simulink model "Hvac_control"  (R2021a)
settings: Solver=ode45  StartTime=0  StopTime=Tf  FixedStep=Ts  RelTol=1e-3
values from neighbouring files (symbols this model uses):
  b = []    [control_predictivo.m]
  Ts = 600    [p2.m]
undefined symbols (not defined in the file or in its folder): a, g
libraries: simulink x2
settings Model: Creator=rober  LastModifiedBy=sebag
settings SolverCC: AlgebraicLoopSolver=TrustRegion
settings DataIOCC: ReturnWorkspaceOutputs=off
settings OptimizationCC: LifeSpan=inf
settings DebuggingCC: SFMachineParentedDataDiag=warning  ArithmeticOperatorsInVariantConditions=warning
settings SFSimCC: CustomCodeUndefinedFunction=UseInterfaceOnly
settings CodeAppCC: StateflowObjectComments=on

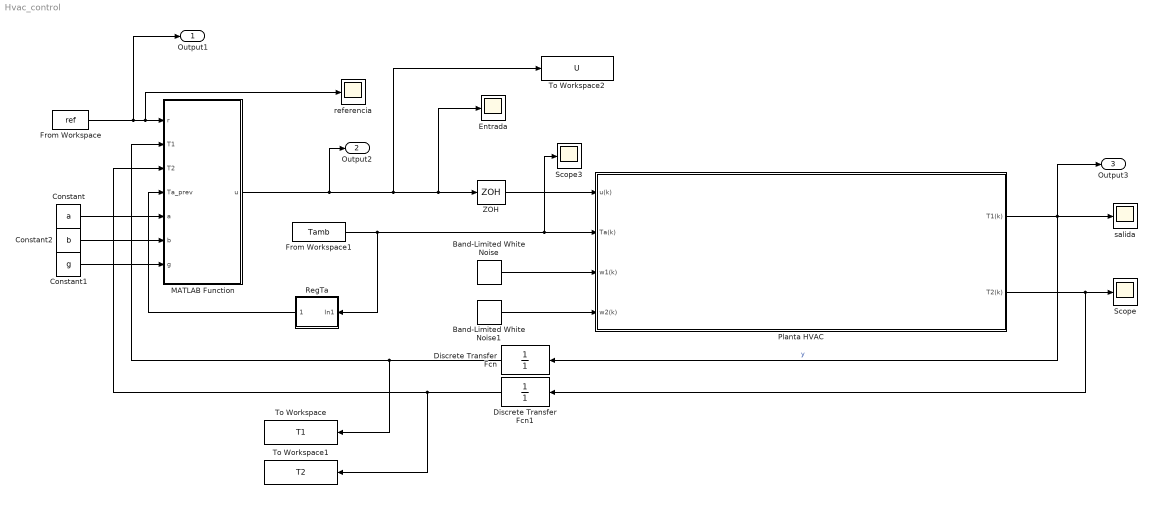
== system Hvac_control ==
  Band-Limited White Noise : simulink/Sources/Band-Limited White Noise  Cov=[0.001]  Ts=Ts  seed=[23341]
  Band-Limited White Noise1 : simulink/Sources/Band-Limited White Noise  Cov=[0.001]  Ts=Ts  seed=[23341]
  Constant : Constant  Value=a
  Constant1 : Constant  Value=g
  Constant2 : Constant  Value=b
  Discrete Transfer Fcn : DiscreteTransferFcn  Denominator=[1]  SampleTime=Ts
  Discrete Transfer Fcn1 : DiscreteTransferFcn  Denominator=[1]  SampleTime=Ts
  Entrada : Scope
  From Workspace : FromWorkspace  VariableName=ref  SampleTime=Ts
  From Workspace1 : FromWorkspace  VariableName=Tamb
  MATLAB Function : MATLAB Function  TreatAsAtomicUnit=on
  Planta HVAC : Subsystem
      mask Display: image('Planta_HVAC.jpg')
  RegTa : Subsystem
  Scope : Scope
  Scope3 : Scope
  To Workspace : ToWorkspace  VariableName=T1  SampleTime=-1
      settings: Save2DSignal=2-D array (concatenate along first dimension)
  To Workspace1 : ToWorkspace  VariableName=T2  SampleTime=Ts
      settings: Save2DSignal=2-D array (concatenate along first dimension)
  To Workspace2 : ToWorkspace  VariableName=U  SampleTime=Ts
      settings: Save2DSignal=2-D array (concatenate along first dimension)
  ZOH : ZeroOrderHold  SampleTime=-1
  referencia : Scope
  salida : Scope
  Output1 : Outport  SignalName=ref
  Output2 : Outport  Port=2  SignalName=u  PortDimensions=[1]
  Output3 : Outport  Port=3  SignalName=y  PortDimensions=[1]
  wires:
  From Workspace1/1 -> Scope3/1, Planta HVAC/2(Ta(k)), RegTa/1(In1)
  Band-Limited White Noise/1 -> Planta HVAC/3(w1(k))
  Band-Limited White Noise1/1 -> Planta HVAC/4(w2(k))
  From Workspace/1 -> Output1/1, referencia/1, MATLAB Function/1(r)
  Planta HVAC/2(T2(k)) -> Discrete Transfer Fcn1/1, Scope/1
  RegTa/1(Ta_prev) -> MATLAB Function/4(Ta_prev)
  Planta HVAC/1(T1(k)) -> Discrete Transfer Fcn/1, salida/1, Output3/1  "y"
  Discrete Transfer Fcn1/1 -> To Workspace1/1, MATLAB Function/3(T2)
  Discrete Transfer Fcn/1 -> MATLAB Function/2(T1), To Workspace/1
  Constant/1 -> MATLAB Function/5(a)
  Constant1/1 -> MATLAB Function/7(g)
  Constant2/1 -> MATLAB Function/6(b)
  MATLAB Function/1(u) -> To Workspace2/1, Entrada/1, ZOH/1, Output2/1
  ZOH/1 -> Planta HVAC/1(u(k))

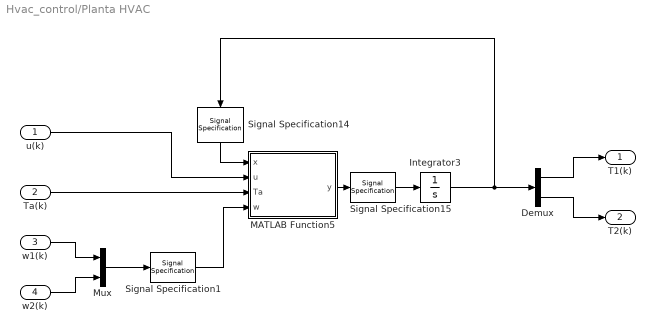
== system Hvac_control/Planta HVAC ==
  u(k) : Inport
  Ta(k) : Inport  Port=2
  w1(k) : Inport  Port=3
  w2(k) : Inport  Port=4
  Demux : Demux  Outputs=2
  Integrator3 : Integrator  InitialCondition=[10.12;10.12]
  MATLAB Function5 : MATLAB Function  TreatAsAtomicUnit=on
  Mux : Mux  Inputs=2
  Signal Specification1 : SignalSpecification  Dimensions=[2,1]  SampleTime=Ts
  Signal Specification14 : SignalSpecification  Dimensions=[2,1]  SampleTime=Ts
  Signal Specification15 : SignalSpecification  Dimensions=[2,1]  SampleTime=Ts
  T1(k) : Outport
  T2(k) : Outport  Port=2
  wires:
  MATLAB Function5/1(y) -> Signal Specification15/1
  Demux/1 -> T1(k)/1
  u(k)/1 -> MATLAB Function5/2(u)
  Ta(k)/1 -> MATLAB Function5/3(Ta)
  Integrator3/1 -> Demux/1, Signal Specification14/1
  Signal Specification14/1 -> MATLAB Function5/1(x)
  Signal Specification15/1 -> Integrator3/1
  Demux/2 -> T2(k)/1
  Mux/1 -> Signal Specification1/1
  w1(k)/1 -> Mux/1
  w2(k)/1 -> Mux/2
  Signal Specification1/1 -> MATLAB Function5/4(w)

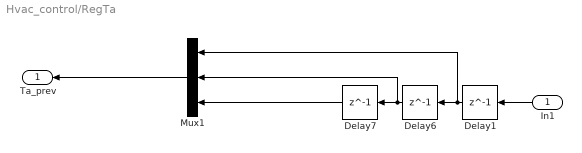
== system Hvac_control/RegTa ==
  In1 : Inport
  Delay1 : Delay  DelayLength=1  SampleTime=Ts
  Delay6 : Delay  DelayLength=1  SampleTime=Ts
  Delay7 : Delay  DelayLength=1  SampleTime=Ts
  Mux1 : Mux  Inputs=3
  Ta_prev : Outport  PortDimensions=[1 3]
  wires:
  In1/1 -> Delay1/1
  Delay6/1 -> Mux1/2, Delay7/1
  Delay7/1 -> Mux1/3
  Mux1/1 -> Ta_prev/1
  Delay1/1 -> Mux1/1, Delay6/1

== matlab function Hvac_control/MATLAB Function ==
  data: r input; T1 input size=[1]; T2 input size=[1]; Ta_prev input size=[1 3]; u output; a input; b input; g input
function u = control(r,T1,T2,Ta_prev, a, b, g)
coder.extrinsic('controller')
u = zeros(1,1);
u = controller(r, T1, T2, Ta_prev, a, b, g);
end

== matlab function Hvac_control/Planta HVAC/MATLAB Function5 ==
  data: x input; u input; y output; Ta input; w input
function y = fcn(x,u,Ta,w)
%% Parametros
c1=2.508*10^6;
c2=4.636*10^7;
cp=1012;
R=1.7*10^(-3);
Ra=1.3*10^(-3);
delta=0.7;
DeltaT=13;
%% Constantes
a1=(cp*(1-delta))/c1;
a2=1/(R*c1);
a3=1/(Ra*c1);
a4=(DeltaT*cp)/c1;
a5=1/c1;
a6=1/(R*c2);
a7=1/c2;
%% Calculo del sistema
xdot=zeros(2,1);
xdot(1)=a1*(Ta-x(1))*u+a2*(x(2)-x(1))+a3*(Ta-x(1))+a4*u+a5*w(1);
xdot(2)=a6*(x(1)-x(2))+a7*w(2);
y = xdot;
